simulink model "Power_converter"  (R2019b)
settings: Solver=VariableStepAuto  StartTime=0.0  StopTime=6  RelTol=1e-3
model workspace (MAT data in the model file):
  Cripple1 = 0.1
  indripple = Simulink.Parameter
  indripple.Value = 0.001
  indripple.DataType = 'auto'
  indripple.DocUnits = 'H'
  indripple.Dimensions = [1 1]
undefined symbols (not defined in the file): sigbuilder_block
libraries: powerlib x38, powerlib_meascontrol x2, simulink x1
settings Model: OrderedModelArguments=off  Creator=Nicholas  LastModifiedBy=Nicholas
settings SolverCC: ZeroCrossAlgorithm=Adaptive
settings DataIOCC: ReturnWorkspaceOutputs=off
settings DebuggingCC: IgnoredZcDiagnostic=none

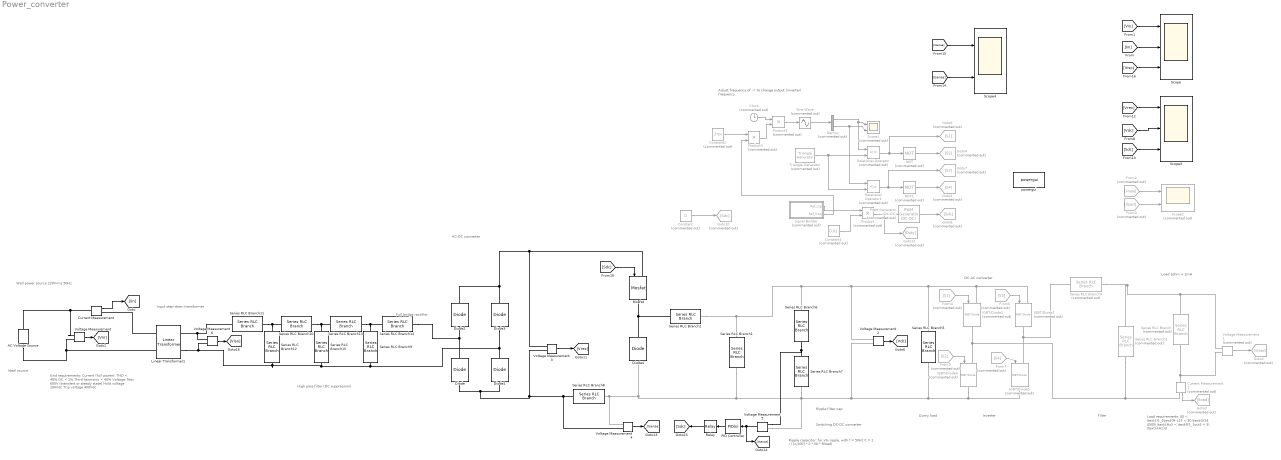
== system Power_converter ==
  note: Wall power source
      | 220Vrms 50Hz
  note: AC-DC converter
  note: Load
      | 1ohm + 1mH
  note: Load requirements:
      | $0 < \text{I}_{\text{R-L}} < 30 \text{A}$
      | $500\ \text{Hz} < \text{f}_{out} < 5\ \text{kHz}$
  note: Grid requirements:
      | Current (full power):
      | THD < 48%
      | DC < 1%
      | Third harmonic < 40%
      |
      | Voltage:
      | Max 600V (transient or steady state)
      | Hold voltage 200Vdc
      | Trip voltage 400Vdc
  note: DC-AC converter
  note: Full bridge rectifier
  note: Switching DC-DC converter
  note: Inverter
  note: Ideal source
  note: Adjust frequency of ->
      | to change output (inverter) frequency.
  note: Filter
  note: Ripple capacitor:
      | for x% ripple, with f = 50Hz
      | C = 1 / ( [x/100] * 2 * 50 * Rload)
  note: Dumy load
  note: Ripple filter cap
  note: Input step-down transformer
  note: High pass filter (DC suppression)
  AC Voltage Source : powerlib/Electrical Sources/AC Voltage Source  Amplitude=220*sqrt(2)  Phase=0  Frequency=50  SampleTime=0  Measurements=None  BusType=PQ  Pref=10e3  Qref=0  Qmin=-inf  Qmax=+inf
      settings: SourceProductName=Simscape Electrical
  Clock : Clock  Commented=on
  Constant : Constant  Commented=on  Value=0
  Constant1 : Constant  Commented=on  Value=0.01
  Constant2 : Constant  Commented=on  Value=2*pi
  Current Measurement : powerlib/Measurements/Current Measurement  PhasorSimulation=off  OutputType=Complex  PSBequivalent=0
      settings: SourceProductName=Simscape Electrical
  Current Measurement1 : powerlib/Measurements/Current Measurement  Commented=on  PhasorSimulation=off  OutputType=Complex  PSBequivalent=0
      settings: SourceProductName=Simscape Electrical
  Demux : Demux  Commented=on  Outputs=2
  Diode{,1..4} (5 alike) : powerlib/Power Electronics/Diode  Ron=0.001  Lon=0  Vf=0.8  IC=0  UseSnubber=0  Rs=500  Cs=250e-9  Measurements=off
      settings: SourceProductName=Simscape Electrical
  From2 : From  Commented=on  GotoTag=Vload
  From3 : From  Commented=on  GotoTag=Iload
  From4 : From  Commented=on  GotoTag=S1
  From5 : From  Commented=on  GotoTag=S2
  From6 : From  Commented=on  GotoTag=S3
  From7 : From  Commented=on  GotoTag=S4
  Goto10 : Goto  Commented=on  GotoTag=Sdc
  Goto12 : Goto  Commented=on  GotoTag=Duty
  Goto2 : Goto  Commented=on  GotoTag=Vload
  Goto3 : Goto  Commented=on  GotoTag=Iload
  Goto4 : Goto  Commented=on  GotoTag=S2
  Goto5 : Goto  Commented=on  GotoTag=S4
  Goto7 : Goto  Commented=on  GotoTag=S3
  Goto8 : Goto  Commented=on  GotoTag=Sdc
  Goto9 : Goto  Commented=on  GotoTag=S1
  IGBT/Diode{1..2,4..5} (4 alike) : powerlib/Power Electronics/IGBT//Diode  Commented=on  Ron=1e-3  Rs=1e5  Cs=inf  Measurements=off
      settings: SourceProductName=Simscape Electrical
  Linear Transformer1 : powerlib/Elements/Linear Transformer  UNITS=pu  NominalPower=[ 250e6 50 ]  winding1="[ (220*sqrt(2))  0.002  0.08 ]"  winding2="[ 75  0.002  0.08 ]"  ThreeWindings=off  winding3=[ 315e3 0.002 0.08 ]  RmLm=[ 500 500 ]  Measurements=None  DataType=off
      settings: SourceProductName=Simscape Electrical
  Mosfet : powerlib/Power Electronics/Mosfet  Ron=0.1  Lon=0  Rd=0.01  Vfd=0  IC=0  Rs=1e5  Cs=inf  Measurements=off
      settings: SourceProductName=Simscape Electrical
  NOT : Logic  Commented=on  Operator=NOT  IconShape=distinctive  AllPortsSameDT=off  OutDataTypeStr=boolean
  NOT1 : Logic  Commented=on  Operator=NOT  IconShape=distinctive  AllPortsSameDT=off  OutDataTypeStr=boolean
  PID Controller : simulink/Continuous/PID Controller  Controller=PID  Form=Parallel  TimeDomain=Continuous-time  SampleTime=-1  IntegratorMethod=Forward Euler  FilterMethod=Forward Euler  ControllerParametersSource=internal  P=1  I=0.05  D=0.5  UseFilter=on  N=100  TunerSelectOption=Transfer Function Based (PID Tuner App)  InitialConditionSource=internal  InitialConditionForIntegrator=0  InitialConditionForFilter=0  DifferentiatorICPrevScaledInput=0  ExternalReset=none  TrackingMode=off  Kt=1  LimitOutput=off  UpperSaturationLimit=inf  LowerSaturationLimit=-inf  LinearizeAsGain=on  AntiWindupMode=none  Kb=1  POutMin=[]  POutMax=[]  IOutMin=[]  IOutMax=[]  DOutMin=[]  DOutMax=[]  NOutMin=[]  NOutMax=[]  SumOutMin=[]  SumOutMax=[]  SaturationOutMin=[]  SaturationOutMax=[]  PParamMin=[]  PParamMax=[]  IParamMin=[]  IParamMax=[]  DParamMin=[]  DParamMax=[]  NParamMin=[]  NParamMax=[]  KbParamMin=[]  KbParamMax=[]  KtParamMin=[]  KtParamMax=[]  KbOutMin=[]  KbOutMax=[]  KtOutMin=[]  KtOutMax=[]  IntegratorOutMin=[]  IntegratorOutMax=[]  FilterOutMin=[]  FilterOutMax=[]  SumI1OutMin=[]  SumI1OutMax=[]  SumI2OutMin=[]  SumI2OutMax=[]  SumI3OutMin=[]  SumI3OutMax=[]  SumI4OutMin=[]  SumI4OutMax=[]  SumDOutMin=[]  SumDOutMax=[]  DifferentiatorOutMin=[]  DifferentiatorOutMax=[]  FilterDiffOutCoefMin=[]  FilterDiffOutCoefMax=[]  ReciprocalOutMin=[]  ReciprocalOutMax=[]  SumDenOutMin=[]  SumDenOutMax=[]  SumNumOutMin=[]  SumNumOutMax=[]  DivideOutMin=[]  DivideOutMax=[]  IntegratorContinuousStateAttributes=''  IntegratorStateMustResolveToSignalObject=off  IntegratorRTWStateStorageClass=Auto  FilterContinuousStateAttributes=''  FilterStateMustResolveToSignalObject=off  FilterRTWStateStorageClass=Auto  ParallelPVariant=InternalParameters  IdealPVariant=Disabled  IVariant=InternalParameters  DVariant=InternalParameters  IntegratorVariant=Continuous  SatVariant=Disabled  AWVariant=Passthrough  PCopyVariant=Disabled  TRVariant=Disabled  FdbkBlocksVariant=Forward  IdealPFdbkVariant=Disabled  SatFdbkVariant=Disabled  DerivativeFilterVariant=ContFilter  NVariant=InternalParameters  NCopyVariant=Disabled  FilterICVariant=InternalICsFilter  IntegratorICVariant=InternalICs  ExternalResetVariant=Disabled  TRSumVariant=Passthrough  SumFdbkVariant=Disabled  SumVariant=Sum_PID
  PWM Generator (DC-DC) : powerlib_meascontrol/Pulse & Signal Generators/PWM Generator (DC-DC)  Commented=on  Fsw=5000  Ts=0
      settings: SourceProductName=Simscape Electrical
  Product : Product  Commented=on
  Product3 : Product  Commented=on
  Product4 : Product  Commented=on
  Relational Operator : RelationalOperator  Commented=on  Operator=<=  OutDataTypeStr=boolean  RndMeth=Simplest
  Relational Operator1 : RelationalOperator  Commented=on  Operator=<=  OutDataTypeStr=boolean  RndMeth=Simplest
  Relay : Relay  OnSwitchValue=41  OffSwitchValue=39  OnOutputValue=0  OffOutputValue=1
  Scope : Scope  NumInputPorts=3
  Scope1 : Scope  Commented=on  NumInputPorts=2
  Scope2 : Scope  Commented=on  NumInputPorts=2
  Scope3 : Scope  NumInputPorts=3
  Scope4 : Scope  NumInputPorts=2
  Series RLC Branch : powerlib/Elements/Series RLC Branch  Commented=on  LConnTagsString=__new0  RConnTagsString=__new0  BranchType=RL  Resistance=1  Inductance=0.1e-3  SetiL0=off  InitialCurrent=0  Capacitance=1e-6  Setx0=off  InitialVoltage=0  Measurements=None
      settings: SourceProductName=Simscape Electrical
  Series RLC Branch1 : powerlib/Elements/Series RLC Branch  LConnTagsString=__new0  RConnTagsString=__new0  BranchType=C  Resistance=1  Inductance=0.1e-3  SetiL0=off  InitialCurrent=0  Capacitance=0.002  Setx0=off  InitialVoltage=0  Measurements=None
      settings: SourceProductName=Simscape Electrical
  Series RLC Branch10 : powerlib/Elements/Series RLC Branch  LConnTagsString=__new0  RConnTagsString=__new0  BranchType=C  Resistance=1  Inductance=0.1e-3  SetiL0=off  InitialCurrent=0  Capacitance=0.000043  Setx0=off  InitialVoltage=0  Measurements=None
      settings: SourceProductName=Simscape Electrical
  Series RLC Branch11 : powerlib/Elements/Series RLC Branch  LConnTagsString=__new0  RConnTagsString=__new0  BranchType=C  Resistance=1  Inductance=0.1e-3  SetiL0=off  InitialCurrent=0  Capacitance=0.000180  Setx0=off  InitialVoltage=0  Measurements=None
      settings: SourceProductName=Simscape Electrical
  Series RLC Branch12 : powerlib/Elements/Series RLC Branch  LConnTagsString=__new0  RConnTagsString=__new0  BranchType=L  Resistance=1  Inductance=0.160  SetiL0=off  InitialCurrent=0  Capacitance=100e-3  Setx0=off  InitialVoltage=0  Measurements=None
      settings: SourceProductName=Simscape Electrical
  Series RLC Branch13 : powerlib/Elements/Series RLC Branch  LConnTagsString=__new0  RConnTagsString=__new0  BranchType=C  Resistance=1  Inductance=0.1e-3  SetiL0=off  InitialCurrent=0  Capacitance=0.000043  Setx0=off  InitialVoltage=0  Measurements=None
      settings: SourceProductName=Simscape Electrical
  Series RLC Branch14 : powerlib/Elements/Series RLC Branch  LConnTagsString=__new0  RConnTagsString=__new0  BranchType=C  Resistance=1  Inductance=0.1e-3  SetiL0=off  InitialCurrent=0  Capacitance=0.000180  Setx0=off  InitialVoltage=0  Measurements=None
      settings: SourceProductName=Simscape Electrical
  Series RLC Branch15 : powerlib/Elements/Series RLC Branch  LConnTagsString=__new0  RConnTagsString=__new0  BranchType=L  Resistance=1  Inductance=0.100  SetiL0=off  InitialCurrent=0  Capacitance=100e-3  Setx0=off  InitialVoltage=0  Measurements=None
      settings: SourceProductName=Simscape Electrical
  Series RLC Branch2 : powerlib/Elements/Series RLC Branch  LConnTagsString=__new0  RConnTagsString=__new0  BranchType=L  Resistance=1  Inductance=0.1e-3  SetiL0=off  InitialCurrent=0  Capacitance=0.002  Setx0=off  InitialVoltage=0  Measurements=None
      settings: SourceProductName=Simscape Electrical
  Series RLC Branch3 : powerlib/Elements/Series RLC Branch  Commented=on  LConnTagsString=__new0  RConnTagsString=__new0  BranchType=C  Resistance=1  Inductance=0.1e-3  SetiL0=off  InitialCurrent=0  Capacitance=100e-3  Setx0=off  InitialVoltage=0  Measurements=None
      settings: SourceProductName=Simscape Electrical
  Series RLC Branch4 : powerlib/Elements/Series RLC Branch  Commented=on  LConnTagsString=__new0  RConnTagsString=__new0  BranchType=L  Resistance=1  Inductance=0.1e-3  SetiL0=off  InitialCurrent=0  Capacitance=100e-3  Setx0=off  InitialVoltage=0  Measurements=None
      settings: SourceProductName=Simscape Electrical
  Series RLC Branch5 : powerlib/Elements/Series RLC Branch  LConnTagsString=__new0  RConnTagsString=__new0  BranchType=R  Resistance=50  Inductance=0.1e-3  SetiL0=off  InitialCurrent=0  Capacitance=0.002  Setx0=off  InitialVoltage=0  Measurements=None
      settings: SourceProductName=Simscape Electrical
  Series RLC Branch6 : powerlib/Elements/Series RLC Branch  LConnTagsString=__new0  RConnTagsString=__new0  BranchType=R  Resistance=1E6  Inductance=0.1e-3  SetiL0=off  InitialCurrent=0  Capacitance=0.002  Setx0=off  InitialVoltage=0  Measurements=None
      settings: SourceProductName=Simscape Electrical
  Series RLC Branch7 : powerlib/Elements/Series RLC Branch  LConnTagsString=__new0  RConnTagsString=__new0  BranchType=R  Resistance=1E6  Inductance=0.1e-3  SetiL0=off  InitialCurrent=0  Capacitance=0.002  Setx0=off  InitialVoltage=0  Measurements=None
      settings: SourceProductName=Simscape Electrical
  Series RLC Branch8 : powerlib/Elements/Series RLC Branch  LConnTagsString=__new0  RConnTagsString=__new0  BranchType=R  Resistance=0.01  Inductance=0.1e-3  SetiL0=off  InitialCurrent=0  Capacitance=0.002  Setx0=off  InitialVoltage=0  Measurements=None
      settings: SourceProductName=Simscape Electrical
  Series RLC Branch9 : powerlib/Elements/Series RLC Branch  LConnTagsString=__new0  RConnTagsString=__new0  BranchType=L  Resistance=1  Inductance=0.160  SetiL0=off  InitialCurrent=0  Capacitance=100e-3  Setx0=off  InitialVoltage=0  Measurements=None
      settings: SourceProductName=Simscape Electrical
  Signal Builder : Subsystem  Tag=STV Subsys  Commented=on  LoadFcn=sigbuilder_block('load');  StartFcn=sigbuilder_block('start');  StopFcn=sigbuilder_block('stop');  ClipboardFcn=sigbuilder_block('clipboard');  mask(Sigbuilder block){tuvar=[0:10]}
      mask help: Simulink:masks:SigbuilderBlock_MD
      mask init:
      | if ~strcmp(get_param(bdroot(gcbh),'SimulationStatus'),'stopped') tuvar = sigbuilder_block('maskInit'); end
      settings: CopyFcn=sigbuilder_block('copy');  DeleteFcn=sigbuilder_block('delete');  ModelCloseFcn=sigbuilder_block('modelClose');  PreSaveFcn=sigbuilder_block('preSave');  PauseFcn=sigbuilder_block('pause');  ContinueFcn=sigbuilder_block('continue');  NameChangeFcn=sigbuilder_block('namechange');  OpenFcn=sigbuilder_block('open',[581.25 327.75 550.5 318.75 ]);  CloseFcn=sigbuilder_block('close');
      mask Display: plot(0, 0, 100, 100,[2, 2, 32, 32, 2], [68, 8, 8, 68, 68],[32, 2], [38, 38], [32, 19, 2],[53, 60, 44], [32, 17, 17, 2],[16, 16, 31, 31]);txt = getActiveGroup(gcbh);text(2, 100, txt,'verticalAlignment', 'top');
  Sine Wave : Sin  Commented=on  TimeSource=Use external signal  Amplitude=[1 1]  Bias=[0 0]  Frequency=[1 1]  Phase=[0 pi]  SampleTime=0
  Triangle Generator : powerlib_meascontrol/Pulse & Signal Generators/Triangle Generator  Commented=on  Freq=1e4  Phase=0  Ts=0
      settings: SourceProductName=Simscape Electrical
  Voltage Measurement{,2..6} (6 alike) : powerlib/Measurements/Voltage Measurement  PhasorSimulation=off  OutputType=Complex  PSBequivalent=0
      settings: SourceProductName=Simscape Electrical
  Voltage Measurement1 : powerlib/Measurements/Voltage Measurement  Commented=on  PhasorSimulation=off  OutputType=Complex  PSBequivalent=0
      settings: SourceProductName=Simscape Electrical
  powergui : powerlib/powergui  Priority=1  SimulationMode=Continuous  SampleTime=50e-6  frequency=60  Iterations=50  frequencyindice=50  Pbase=100e6  ErrMax=1e-4  UnitsV=kV  UnitsW=MW  buscounter=0  FunctionMessages=off  echomessages=off  EnableUseOfTLC=off  CurrentSourceSwitches=off  DisableSnubberDevices=off  DisableRonSwitches=off  DisableVfSwitches=off  DisplayEquations=off  AutomaticDiscreteSolvers=off  SolverType=Tustin/Backward Euler (TBE)  Interpol=off  ExternalGateDelay=off  methode=off  Ts=100  x0status=blocks  SPID=on  SwTol=0  HookPort=off  NonlinearTolerance=1e-4  nMaxIteration=100  ContinueOnMaxIteration=off  RestoreLinks=warning  ResistiveCurrentMeasurement=off  Frange=[0:2:500]  Ylog=off  Xlog=on  ShowGrid=off  save=off  variable=ZData  structure=ScopeData  ZoomFFT=on  StartTime=0.0  cycles=1  DisplayStyle=1  fundamental=50  FreqAxis=off  MaxFrequency=1000  frequencyindicesteady=1  RmsSteady=1  display=off
      settings: SourceProductName=Simscape Electrical
  wires:
  Voltage Measurement/1 -> [Vin]
  Current Measurement/1 -> [Iin]
  Voltage Measurement1/1 -> Goto2/1
  [Iin] -> Scope/2
  [Vin] -> Scope/1
  Current Measurement1/1 -> Goto3/1
  From6/1 -> IGBT/Diode2/1
  From5/1 -> IGBT/Diode4/1
  From4/1 -> IGBT/Diode1/1
  From7/1 -> IGBT/Diode5/1
  Relational Operator1/1 -> Goto7/1, NOT1/1
  Triangle Generator/1 -> Relational Operator1/2, Relational Operator/2
  Sine Wave/1 -> Demux/1
  Relational Operator/1 -> Goto9/1, NOT/1
  NOT/1 -> Goto4/1
  Demux/2 -> Relational Operator1/1, Scope1/2
  Demux/1 -> Relational Operator/1, Scope1/1
  NOT1/1 -> Goto5/1
  Voltage Measurement2/1 -> [Vdc]
  PWM Generator (DC-DC)/1 -> Goto8/1
  Signal Builder/1(Ref_sig) -> Product/1
  Constant1/1 -> Product/2
  Product/1 -> Goto12/1, PWM Generator (DC-DC)/1
  Product3/1 -> Sine Wave/1
  Clock/1 -> Product3/1
  Signal Builder/2(Ref_freq) -> Product4/2
  Constant2/1 -> Product4/1
  Product4/1 -> Product3/2
  From2/1 -> Scope2/1
  From3/1 -> Scope2/2
  Constant/1 -> Goto10/1
  [Sdc] -> Mosfet/1
  [Vdc] -> Scope3/2
  Voltage Measurement3/1 -> [Vrec]
  [Vrec] -> Scope3/1
  [Sdc] -> Scope3/3
  Voltage Measurement4/1 -> [Isense]
  [Isense] -> Scope4/2
  [Vsense] -> Scope4/1
  Relay/1 -> [Sdc]
  Voltage Measurement5/1 -> PID Controller/1, [Vsense]
  PID Controller/1 -> Relay/1
  Voltage Measurement6/1 -> [Viso]
  [Viso] -> Scope/3
  connections:
  Voltage Measurement/LConn1 -- AC Voltage Source/RConn1 -- Current Measurement/LConn1
  Diode2/RConn1 -- Voltage Measurement3/LConn1 -- Mosfet/LConn1 -- Diode3/RConn1
  Current Measurement1/LConn1 -- Voltage Measurement1/LConn2 -- Series RLC Branch/RConn1
  IGBT/Diode4/RConn1 -- Series RLC Branch5/RConn1 -- Voltage Measurement2/LConn2 -- Voltage Measurement5/LConn2 -- Series RLC Branch7/RConn1 -- Voltage Measurement4/LConn2 -- Series RLC Branch8/LConn1 -- Diode4/LConn1 -- Series RLC Branch1/RConn1 -- IGBT/Diode5/RConn1
  Diode/RConn1 -- Series RLC Branch14/RConn1 -- Diode2/LConn1
  IGBT/Diode2/LConn1 -- IGBT/Diode1/LConn1 -- Series RLC Branch5/LConn1 -- Series RLC Branch6/LConn1 -- Series RLC Branch2/RConn1 -- Series RLC Branch1/LConn1 -- Voltage Measurement2/LConn1
  IGBT/Diode2/RConn1 -- Series RLC Branch4/LConn1 -- IGBT/Diode5/LConn1
  Linear Transformer1/RConn2 -- Voltage Measurement6/LConn2 -- Diode1/RConn1 -- Diode3/LConn1 -- Series RLC Branch9/RConn1 -- Series RLC Branch15/RConn1 -- Series RLC Branch12/RConn1
  IGBT/Diode1/RConn1 -- Series RLC Branch3/RConn1 -- Current Measurement1/RConn1 -- IGBT/Diode4/LConn1
  Voltage Measurement1/LConn1 -- Series RLC Branch4/RConn1 -- Series RLC Branch3/LConn1 -- Series RLC Branch/LConn1
  Series RLC Branch2/LConn1 -- Mosfet/RConn1 -- Diode4/RConn1
  Series RLC Branch6/RConn1 -- Voltage Measurement5/LConn1 -- Series RLC Branch7/LConn1
  Diode/LConn1 -- Voltage Measurement4/LConn1 -- Series RLC Branch8/RConn1 -- Voltage Measurement3/LConn2 -- Diode1/LConn1
  AC Voltage Source/LConn1 -- Linear Transformer1/LConn2 -- Voltage Measurement/LConn2
  Series RLC Branch15/LConn1 -- Series RLC Branch10/RConn1 -- Series RLC Branch13/LConn1
  Series RLC Branch12/LConn1 -- Series RLC Branch11/RConn1 -- Series RLC Branch10/LConn1
  Series RLC Branch9/LConn1 -- Series RLC Branch13/RConn1 -- Series RLC Branch14/LConn1
  Series RLC Branch11/LConn1 -- Voltage Measurement6/LConn1 -- Linear Transformer1/RConn1
  Linear Transformer1/LConn1 -- Current Measurement/RConn1

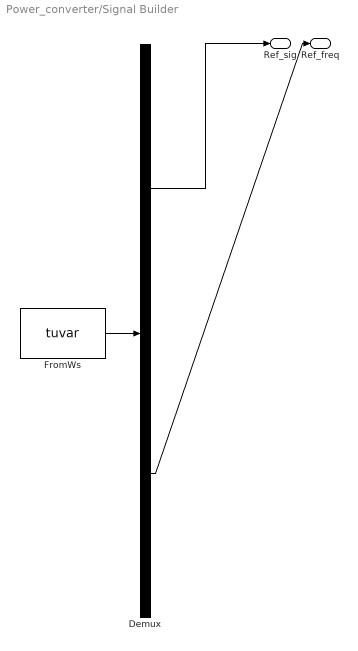
== system Power_converter/Signal Builder ==
  Demux : Demux  Tag=STV Demux  Outputs=2
  FromWs : FromWorkspace  Tag=STV FromWs  VariableName=tuvar  SampleTime=0
      SigBuilderData=|
      | common.afterFinalStr = 'Extrapolate'
      | common.sampleTime = 0
      | dataSet.timeRange = [0 10]
      | dataSet.name = 'Group 1'
      | sbobj.Groups.Name = 'Group 1'
      | sbobj.Groups.Signals(1).Name = 'Ref_sig'
      | sbobj.Groups.Signals(1).XData = [0 1 1 3 3 5 5.5 6 6 10]
      | sbobj.Groups.Signals(1).YData = [3 3 20 20 10 10 18 18 0 0]
      | sbobj.Groups.Signals(2).Name = 'Ref_freq'
      | sbobj.Groups.Signals(2).XData = [0 1 1 3 3 10]
      | sbobj.Groups.Signals(2).YData = [500 500 5000 5000 1000 1000]
  Ref_sig : Outport  Tag=STV Outport
  Ref_freq : Outport  Tag=STV Outport  Port=2
  wires:
  Demux/1 -> Ref_sig/1
  FromWs/1 -> Demux/1
  Demux/2 -> Ref_freq/1
